simulink model "model_NNMPC"  (R2025a)
settings: Solver=VariableStepAuto  StartTime=0.0  StopTime=200000  RelTol=1e-4
values from neighbouring files (symbols this model uses):
  T0 = 320    [init_params.m]
  Tc0 = 298    [init_params.m]
settings Model: Creator=thapl  LastModifiedBy=thapl
settings DataIOCC: SaveFormat=Array
settings OptimizationCC: ReuseModelBlockBuffer=off
settings RTWCC: GPUComputeCapability=3.5

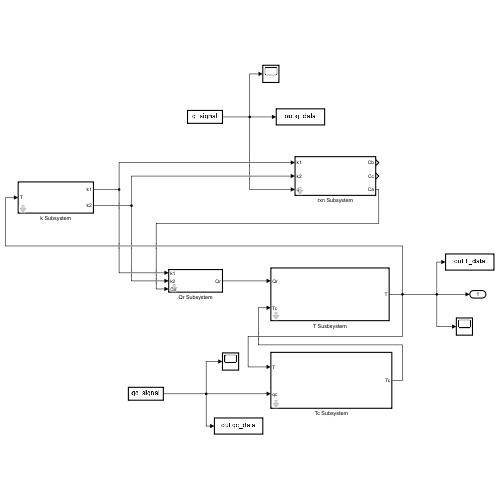
[thumbnail: Simulink's stored preview of the top-level diagram]
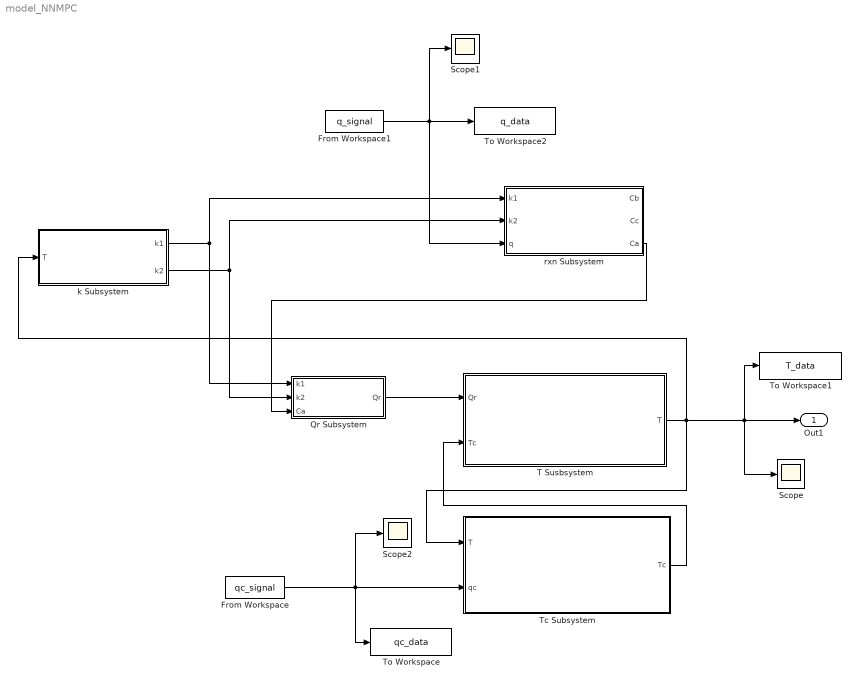
== system model_NNMPC ==
  From Workspace : FromWorkspace  VariableName=qc_signal
  From Workspace1 : FromWorkspace  VariableName=q_signal
  Qr Subsystem : Subsystem  mask{V=0.23, dH1=-8.6e4, dH2=-1.82e4}
      mask prompts: V "Reactor Volume (V)"; dH1 "Enthapy of Rxn1 (dH1)"; dH2 "Enthalpy of Rxn2 (dH2)"
  Scope : Scope
      settings: ActiveDisplayYMinimum=300.31208265781891  ActiveDisplayYMaximum=320.01283178936956
  Scope1 : Scope
      settings: ActiveDisplayYMinimum=0.039296210816251953  ActiveDisplayYMaximum=0.040424018972038171  DataLoggingVariableName=ScopeData2
  Scope2 : Scope
      settings: ActiveDisplayYMinimum=-0.0043  ActiveDisplayYMaximum=0.04488
  T Susbsystem : Subsystem  mask{q=0.015, V=0.23, Tf=311, A=1.51, u=42.8, rho=1020, Cp=4.02}
      mask prompts: q "Reactor Flow rate (q)"; V "Reactor Volume (V)"; Tf "Inlet Fluid Temp (Tf)"; A "Contact Area (A)"; u "HTC (u)"; rho "Fluid Density (rho)"; Cp "Specific Heat capactiy (Cp)"
  Tc Subsystem : Subsystem  mask{Vc=0.21, Tcf=292, A=1.51, u=42.8, Cpc=4.182, rhoc=998}
      mask prompts: Vc "Jacket Volume (Vc)"; Tcf "Inlet Cooling Fluid Tempreture (Tcf)"; A "Contact Area (A)"; u "HTC"; Cpc "Specidic Heat Capacity of cooling fluid (Cpc)"; rhoc "Cooling Fluid Density (rhoc)"
  To Workspace : ToWorkspace  VariableName=qc_data  SaveFormat=Timeseries  SampleTime=-1
      settings: Save2DSignal=2-D array (concatenate along first dimension)
  To Workspace1 : ToWorkspace  VariableName=T_data  SaveFormat=Timeseries  SampleTime=-1
      settings: Save2DSignal=2-D array (concatenate along first dimension)
  To Workspace2 : ToWorkspace  VariableName=q_data  SaveFormat=Timeseries  SampleTime=-1
  k Subsystem : Subsystem
      mask DialogControl Control2 Prompt: Text
  rxn Subsystem : Subsystem
      mask DialogControl Control2 Prompt: Reactor
  Out1 : Outport
  wires:
  Tc Subsystem/1(Tc) -> T Susbsystem/2(Tc)
  T Susbsystem/1(T) -> k Subsystem/1(T), Scope/1, To Workspace1/1, Out1/1, Tc Subsystem/1(T)
  Qr Subsystem/1(Qr) -> T Susbsystem/1(Qr)
  From Workspace/1 -> Scope2/1, To Workspace/1, Tc Subsystem/2(qc)
  rxn Subsystem/3(Ca) -> Qr Subsystem/3(Ca)
  k Subsystem/1(k1) -> rxn Subsystem/1(k1), Qr Subsystem/1(k1)
  k Subsystem/2(k2) -> rxn Subsystem/2(k2), Qr Subsystem/2(k2)
  From Workspace1/1 -> Scope1/1, To Workspace2/1, rxn Subsystem/3(q)

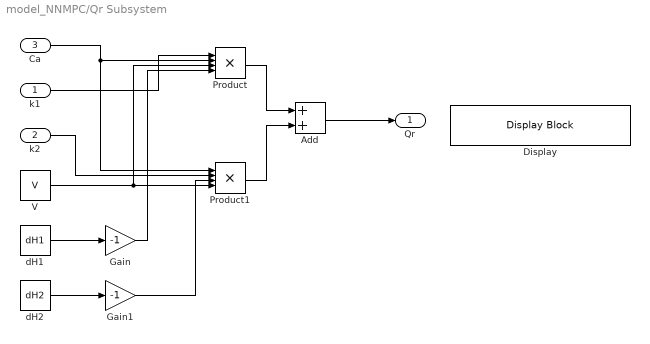
== system model_NNMPC/Qr Subsystem ==
  k1 : Inport
  k2 : Inport  Port=2
  Ca : Inport  Port=3
  Add : Sum
  Display : DisplayBlock  LabelPosition=Hide  Transparency=1  GridColor=[0.502, 0.502, 0.502]
  Gain : Gain  Gain=-1
  Gain1 : Gain  Gain=-1
  Product : Product  Inputs=4
  Product1 : Product  Inputs=4
  V : Constant  Value=V
  dH1 : Constant  Value=dH1
  dH2 : Constant  Value=dH2
  Qr : Outport
  wires:
  dH1/1 -> Gain/1
  dH2/1 -> Gain1/1
  k1/1 -> Product/1
  V/1 -> Product1/4, Product/3
  Gain/1 -> Product/4
  Ca/1 -> Product1/1, Product/2
  k2/1 -> Product1/2
  Gain1/1 -> Product1/3
  Product/1 -> Add/1
  Product1/1 -> Add/2
  Add/1 -> Qr/1

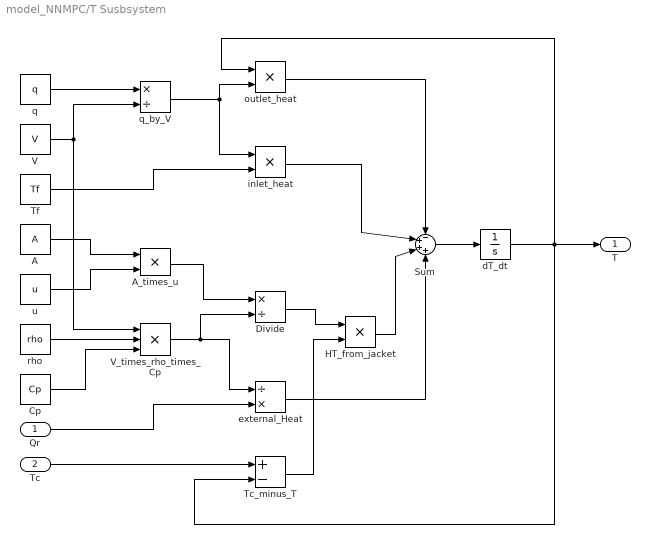
== system model_NNMPC/T Susbsystem ==
  Qr : Inport
  Tc : Inport  Port=2
  A : Constant  Value=A
  A_times_u : Product
  Cp : Constant  Value=Cp
  Divide : Product  Inputs=*/
  HT_from_jacket : Product
  Sum : Sum  Inputs=-+++
  Tc_minus_T : Sum  Inputs=+-
  Tf : Constant  Value=Tf
  V : Constant  Value=V
  V_times_rho_times_Cp : Product  Inputs=3
  dT_dt : Integrator  InitialCondition=T0
  external_Heat : Product  Inputs=/*
  inlet_heat : Product
  outlet_heat : Product
  q : Constant  Value=q
  q_by_V : Product  Inputs=*/
  rho : Constant  Value=rho
  u : Constant  Value=u
  T : Outport
  wires:
  q/1 -> q_by_V/1
  V/1 -> V_times_rho_times_Cp/1, q_by_V/2
  q_by_V/1 -> outlet_heat/2, inlet_heat/1
  Tf/1 -> inlet_heat/2
  A/1 -> A_times_u/1
  u/1 -> A_times_u/2
  rho/1 -> V_times_rho_times_Cp/2
  Cp/1 -> V_times_rho_times_Cp/3
  A_times_u/1 -> Divide/1
  V_times_rho_times_Cp/1 -> external_Heat/1, Divide/2
  Divide/1 -> HT_from_jacket/1
  Tc_minus_T/1 -> HT_from_jacket/2
  Qr/1 -> external_Heat/2
  outlet_heat/1 -> Sum/1
  inlet_heat/1 -> Sum/2
  HT_from_jacket/1 -> Sum/3
  external_Heat/1 -> Sum/4
  Sum/1 -> dT_dt/1
  dT_dt/1 -> outlet_heat/1, T/1, Tc_minus_T/2
  Tc/1 -> Tc_minus_T/1

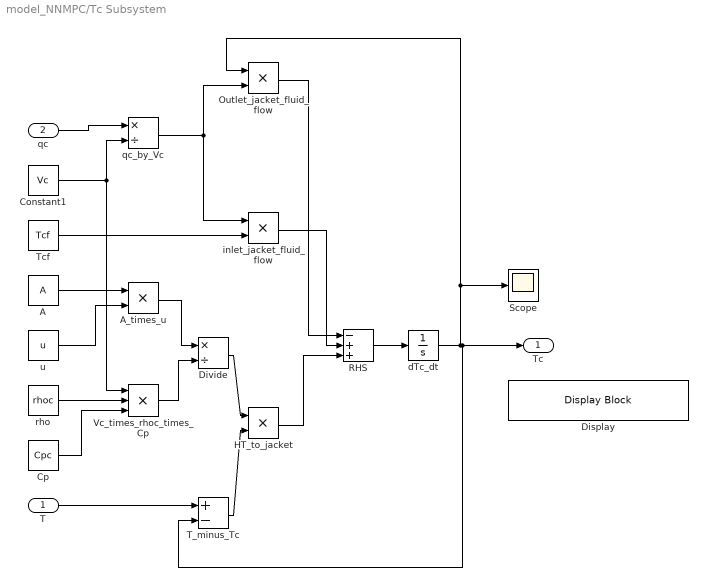
== system model_NNMPC/Tc Subsystem ==
  T : Inport
  qc : Inport  Port=2
  A : Constant  Value=A
  A_times_u : Product
  Constant1 : Constant  Value=Vc
  Cp : Constant  Value=Cpc
  Display : DisplayBlock  LabelPosition=Hide  Transparency=1  GridColor=[0.502, 0.502, 0.502]
  Divide : Product  Inputs=*/
  HT_to_jacket : Product
  Outlet_jacket_fluid_flow : Product
  RHS : Sum  Inputs=-++
  Scope : Scope
      settings: ActiveDisplayYMinimum=291.10857  ActiveDisplayYMaximum=300.98794  DataLoggingVariableName=ScopeData3
  T_minus_Tc : Sum  Inputs=+-
  Tcf : Constant  Value=Tcf
  Vc_times_rhoc_times_Cp : Product  Inputs=3
  dTc_dt : Integrator  InitialCondition=Tc0
  inlet_jacket_fluid_flow : Product
  qc_by_Vc : Product  Inputs=*/
  rho : Constant  Value=rhoc
  u : Constant  Value=u
  Tc : Outport
  wires:
  qc/1 -> qc_by_Vc/1
  Constant1/1 -> Vc_times_rhoc_times_Cp/1, qc_by_Vc/2
  qc_by_Vc/1 -> Outlet_jacket_fluid_flow/2, inlet_jacket_fluid_flow/1
  Tcf/1 -> inlet_jacket_fluid_flow/2
  A/1 -> A_times_u/1
  u/1 -> A_times_u/2
  rho/1 -> Vc_times_rhoc_times_Cp/2
  Cp/1 -> Vc_times_rhoc_times_Cp/3
  A_times_u/1 -> Divide/1
  Vc_times_rhoc_times_Cp/1 -> Divide/2
  T/1 -> T_minus_Tc/1
  Divide/1 -> HT_to_jacket/1
  T_minus_Tc/1 -> HT_to_jacket/2
  HT_to_jacket/1 -> RHS/3
  inlet_jacket_fluid_flow/1 -> RHS/2
  RHS/1 -> dTc_dt/1
  dTc_dt/1 -> Scope/1, Outlet_jacket_fluid_flow/1, Tc/1, T_minus_Tc/2
  Outlet_jacket_fluid_flow/1 -> RHS/1

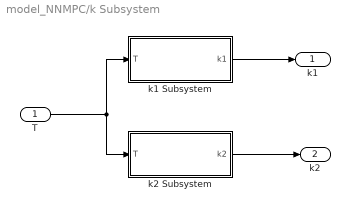
== system model_NNMPC/k Subsystem ==
  T : Inport
  k1 Subsystem : Subsystem  mask{R=8.314, k10=1.55e11, Ea1=9850*8.314}
      mask prompts: R "Universal Gas Constant(R)"; k10 "Pre exponential factor(k10)"; Ea1 "Actvation Energy(Ea1)"
  k2 Subsystem : Subsystem  mask{R=8.314, k20=4.55e25, Ea2=22019*8.314}
      mask prompts: R "Universal Gas Constant(R)"; k20 "Pre exponential factor(k10)"; Ea2 "Actvation Energy(Ea1)"
  k1 : Outport
  k2 : Outport  Port=2
  wires:
  k2 Subsystem/1(k2) -> k2/1
  T/1 -> k2 Subsystem/1(T), k1 Subsystem/1(T)
  k1 Subsystem/1(k1) -> k1/1

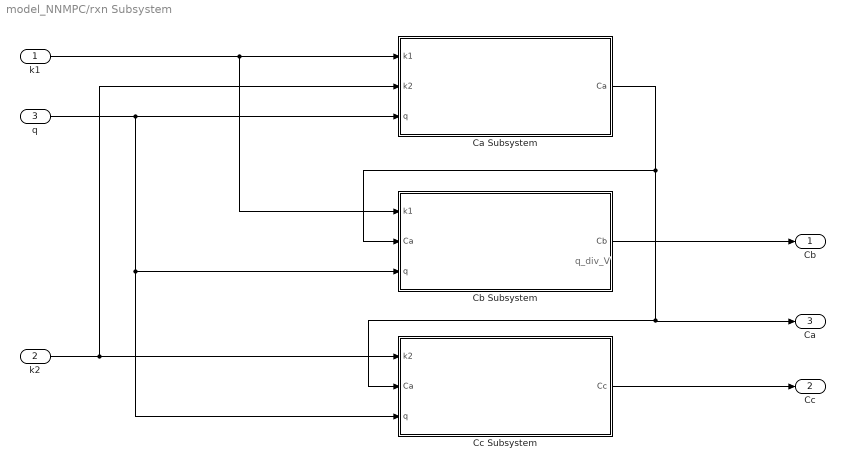
== system model_NNMPC/rxn Subsystem ==
  note: q_div_V
  k1 : Inport
  k2 : Inport  Port=2
  q : Inport  Port=3
  Ca Subsystem : Subsystem  mask{V=0.23, Caf=4.22}
      mask prompts: V "Reactor Volume(V)"; Caf "Feed Conc (Caf)"
  Cb Subsystem : Subsystem  mask{V=0.23, Cbf=0}
      mask prompts: V "Reactor Volume(V)"; Cbf "Feed Conc (Cbf)"
  Cc Subsystem : Subsystem  mask{V=0.23, Ccf=0}
      mask prompts: V "Reactor Volume(V)"; Ccf "Feed Conc (Ccf)"
  Cb : Outport
  Cc : Outport  Port=2
  Ca : Outport  Port=3
  wires:
  k1/1 -> Cb Subsystem/1(k1), Ca Subsystem/1(k1)
  Cc Subsystem/1(Cc) -> Cc/1
  Ca Subsystem/1(Ca) -> Ca/1, Cc Subsystem/2(Ca), Cb Subsystem/2(Ca)
  Cb Subsystem/1(Cb) -> Cb/1
  k2/1 -> Cc Subsystem/1(k2), Ca Subsystem/2(k2)
  q/1 -> Cc Subsystem/3(q), Cb Subsystem/3(q), Ca Subsystem/3(q)

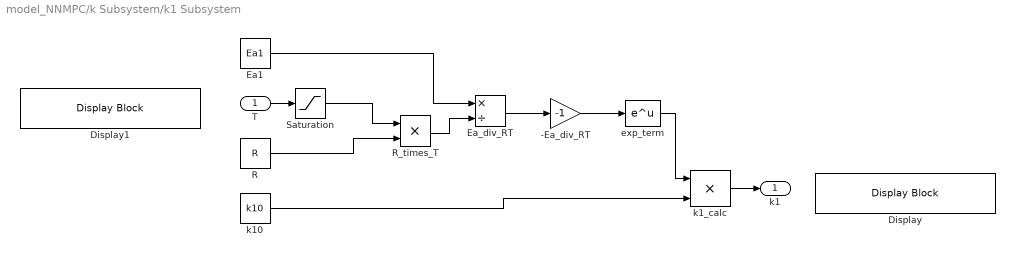
== system model_NNMPC/k Subsystem/k1 Subsystem ==
  T : Inport
  -Ea_div_RT : Gain  Gain=-1
  Display : DisplayBlock  LabelPosition=Hide  Transparency=1  GridColor=[0.502, 0.502, 0.502]
  Display1 : DisplayBlock  LabelPosition=Hide  Transparency=1  GridColor=[0.502, 0.502, 0.502]
  Ea1 : Constant  Value=Ea1
  Ea_div_RT : Product  Inputs=*/
  R : Constant  Value=R
  R_times_T : Product
  Saturation : Saturate  UpperLimit=Inf  LowerLimit=0.001
  exp_term : Math
  k10 : Constant  Value=k10
  k1_calc : Product
  k1 : Outport
  wires:
  R/1 -> R_times_T/2
  Ea1/1 -> Ea_div_RT/1
  R_times_T/1 -> Ea_div_RT/2
  k10/1 -> k1_calc/2
  k1_calc/1 -> k1/1
  Ea_div_RT/1 -> -Ea_div_RT/1
  -Ea_div_RT/1 -> exp_term/1
  exp_term/1 -> k1_calc/1
  T/1 -> Saturation/1
  Saturation/1 -> R_times_T/1

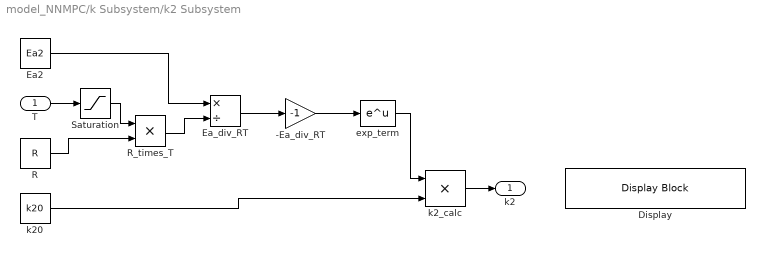
== system model_NNMPC/k Subsystem/k2 Subsystem ==
  T : Inport
  -Ea_div_RT : Gain  Gain=-1
  Display : DisplayBlock  LabelPosition=Hide  Transparency=1  GridColor=[0.502, 0.502, 0.502]
  Ea2 : Constant  Value=Ea2
  Ea_div_RT : Product  Inputs=*/
  R : Constant  Value=R
  R_times_T : Product
  Saturation : Saturate  UpperLimit=Inf  LowerLimit=0.001
  exp_term : Math
  k20 : Constant  Value=k20
  k2_calc : Product
  k2 : Outport
  wires:
  R/1 -> R_times_T/2
  Ea2/1 -> Ea_div_RT/1
  R_times_T/1 -> Ea_div_RT/2
  k20/1 -> k2_calc/2
  k2_calc/1 -> k2/1
  Ea_div_RT/1 -> -Ea_div_RT/1
  -Ea_div_RT/1 -> exp_term/1
  exp_term/1 -> k2_calc/1
  T/1 -> Saturation/1
  Saturation/1 -> R_times_T/1

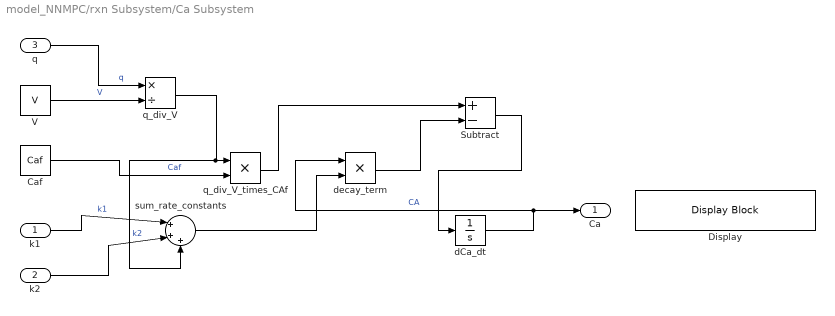
== system model_NNMPC/rxn Subsystem/Ca Subsystem ==
  k1 : Inport
  k2 : Inport  Port=2
  q : Inport  Port=3
  Caf : Constant  Value=Caf
  Display : DisplayBlock  LabelPosition=Hide  Transparency=1  GridColor=[0.502, 0.502, 0.502]
  Subtract : Sum  Inputs=+-
  V : Constant  Value=V  SampleTime=Inf
  dCa_dt : Integrator  InitialCondition=4.22
  decay_term : Product
  q_div_V : Product  Inputs=*/
  q_div_V_times_CAf : Product
  sum_rate_constants : Sum  Inputs=|+++
  Ca : Outport
  wires:
  q/1 -> q_div_V/1  "q"
  V/1 -> q_div_V/2  "V"
  q_div_V/1 -> sum_rate_constants/3, q_div_V_times_CAf/1
  Caf/1 -> q_div_V_times_CAf/2  "Caf"
  k1/1 -> sum_rate_constants/1  "k1"
  k2/1 -> sum_rate_constants/2  "k2"
  sum_rate_constants/1 -> decay_term/2
  dCa_dt/1 -> decay_term/1, Ca/1  "CA"
  decay_term/1 -> Subtract/2
  Subtract/1 -> dCa_dt/1
  q_div_V_times_CAf/1 -> Subtract/1

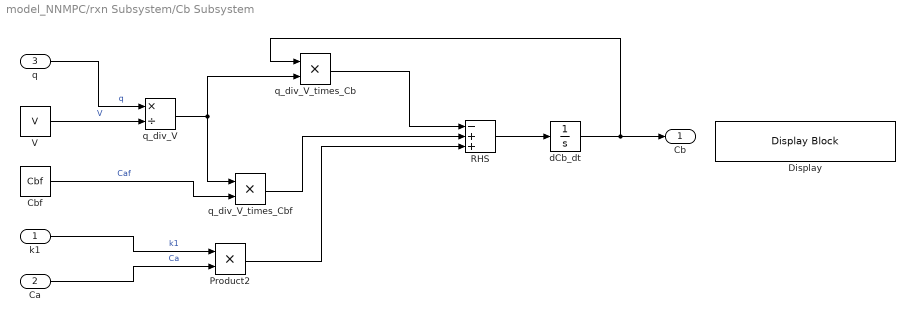
== system model_NNMPC/rxn Subsystem/Cb Subsystem ==
  k1 : Inport
  Ca : Inport  Port=2
  q : Inport  Port=3
  Cbf : Constant  Value=Cbf
  Display : DisplayBlock  LabelPosition=Hide  Transparency=1  GridColor=[0.502, 0.502, 0.502]
  Product2 : Product
  RHS : Sum  Inputs=-++
  V : Constant  Value=V
  dCb_dt : Integrator
  q_div_V : Product  Inputs=*/
  q_div_V_times_Cb : Product
  q_div_V_times_Cbf : Product
  Cb : Outport
  wires:
  q/1 -> q_div_V/1  "q"
  V/1 -> q_div_V/2  "V"
  q_div_V/1 -> q_div_V_times_Cb/2, q_div_V_times_Cbf/1
  Cbf/1 -> q_div_V_times_Cbf/2  "Caf"
  k1/1 -> Product2/1  "k1"
  dCb_dt/1 -> Cb/1, q_div_V_times_Cb/1
  RHS/1 -> dCb_dt/1
  Ca/1 -> Product2/2  "Ca"
  q_div_V_times_Cb/1 -> RHS/1
  q_div_V_times_Cbf/1 -> RHS/2
  Product2/1 -> RHS/3

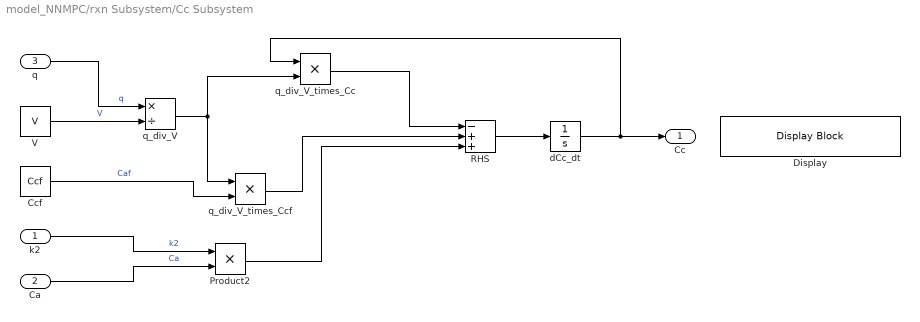
== system model_NNMPC/rxn Subsystem/Cc Subsystem ==
  k2 : Inport
  Ca : Inport  Port=2
  q : Inport  Port=3
  Ccf : Constant  Value=Ccf
  Display : DisplayBlock  LabelPosition=Hide  Transparency=1  GridColor=[0.502, 0.502, 0.502]
  Product2 : Product
  RHS : Sum  Inputs=-++
  V : Constant  Value=V
  dCc_dt : Integrator
  q_div_V : Product  Inputs=*/
  q_div_V_times_Cc : Product
  q_div_V_times_Ccf : Product
  Cc : Outport
  wires:
  q/1 -> q_div_V/1  "q"
  V/1 -> q_div_V/2  "V"
  q_div_V/1 -> q_div_V_times_Cc/2, q_div_V_times_Ccf/1
  Ccf/1 -> q_div_V_times_Ccf/2  "Caf"
  k2/1 -> Product2/1  "k2"
  dCc_dt/1 -> Cc/1, q_div_V_times_Cc/1
  RHS/1 -> dCc_dt/1
  Ca/1 -> Product2/2  "Ca"
  q_div_V_times_Cc/1 -> RHS/1
  q_div_V_times_Ccf/1 -> RHS/2
  Product2/1 -> RHS/3
